simulink model "slip_model_Student"  (Simulink 8.7)
settings: Solver=ode45  StartTime=0.0  StopTime=20  RelTol=1e-3
values from neighbouring files (symbols this model uses):
  AA = [0 1 0 0 0 0; -Veh.kc/Veh.mc -Veh.cc/Veh.mc Veh.kc/Veh.mc Veh.cc/Veh.mc 0 0; 0 0 0 1 0 0; Veh.kc/Veh.mb Veh.cc/Veh.mb -(Veh.kc+Veh.kb)/Veh.mb -(Veh.cc+Veh.cb)/Veh.mb Veh.kb/Veh.mb Veh.cb/Veh.mb; 0 0 0 0 1 0; 0 0 Veh.kb/Veh.mw Veh.cb/Veh.mw -(Veh.kb+Veh.kw)/Veh.mw -(Veh.cb+Veh.cw)/Veh.mw]    [initial.m]
  BB = [0 0; 0 0; 0 0; 0 0; 0 0; Veh.kw/Veh.mw Veh.cw/Veh.mw]    [initial.m]
  CC = [0 0 0 0 -Veh.kw -Veh.cw]    [initial.m]
  DD = [Veh.kw Veh.cw]    [initial.m]
  k_b = 0.6    [Task2b.m]    (also in Task2bLooping.m; Task2c.m = 1; initial.m = 0.2)
  k_t = 0    [Task2b.m]    (also in Task2bLooping.m; Task2c.m = 0.7356; initial.m = 0.23)
  T_max = (Veh.mc+Veh.mb+Veh.mw)*9.81*Veh.r    [initial.m]
undefined symbols (not defined in the file or in its folder): Dri, Veh
libraries: driveline x8, simulink x2
settings Model: Creator=Johannes  LastModifiedBy=Dell
settings DataIOCC: LimitDataPoints=off
settings OptimizationCC: ExpressionDepthLimit=2147483647
settings DebuggingCC: SolverPrmCheckMsg=warning  FcnCallInpInsideContextMsg=UseLocalSettings  StateNameClashWarn=warning
settings GRTTargetCC: CombineOutputUpdateFcns=off  GRTInterface=on

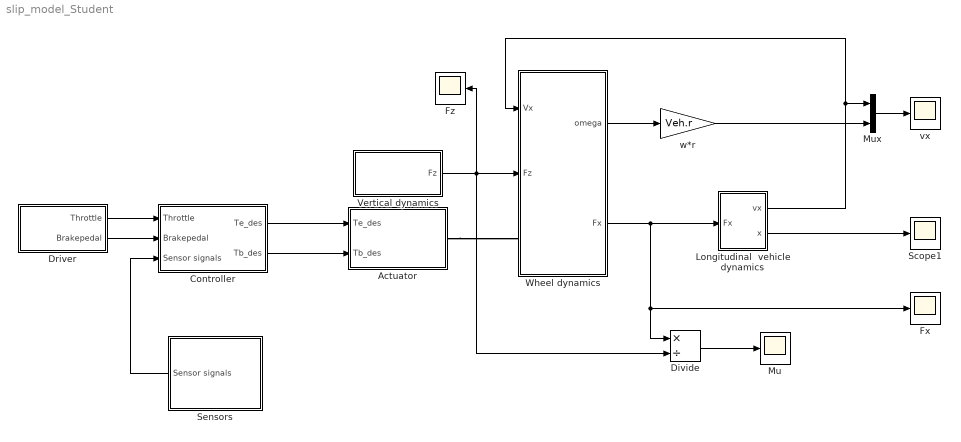
== system slip_model_Student ==
  Actuator : Subsystem
  Controller : Subsystem
  Divide : Product  Inputs=*/
  Driver : Subsystem
  Fx : Scope
  Fz : Scope
  Longitudinal  vehicle dynamics : Subsystem
  "Mu " : Scope
  Mux : Mux  Inputs=2
  Scope1 : Scope
  Sensors : Subsystem
  Vertical dynamics : Subsystem
  Wheel dynamics : Subsystem
  vx : Scope
  w*r : Gain  Gain=Veh.r
  wires:
  Longitudinal  vehicle dynamics/2(x) -> Scope1/1
  Mux/1 -> vx/1
  w*r/1 -> Mux/2
  Wheel dynamics/1(omega) -> w*r/1
  Wheel dynamics/2(Fx) -> Longitudinal  vehicle dynamics/1(Fx), Divide/1, Fx/1
  Vertical dynamics/1(Fz) -> Fz/1, Divide/2, Wheel dynamics/2(Fz)
  Driver/2(Brakepedal) -> Controller/2(Brakepedal)
  Driver/1(Throttle) -> Controller/1(Throttle)
  Controller/1(Te_des) -> Actuator/1(Te_des)
  Controller/2(Tb_des) -> Actuator/2(Tb_des)
  Sensors/1(Sensor signals) -> Controller/3(Sensor signals)
  Longitudinal  vehicle dynamics/1(vx) -> Mux/1, Wheel dynamics/1(Vx)
  Divide/1 -> "Mu "/1
  connections:
  Actuator/RConn1 -- Wheel dynamics/LConn1

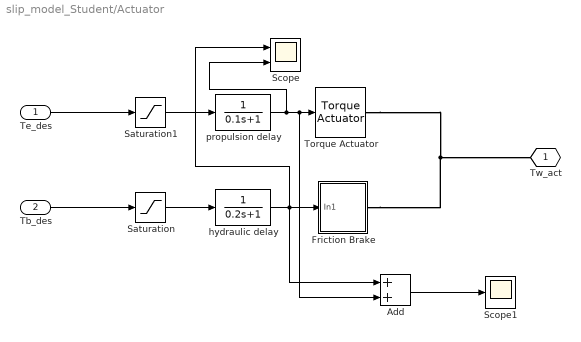
== system slip_model_Student/Actuator ==
  Te_des : Inport
  Tb_des : Inport  Port=2
  Add : Sum
  Friction Brake : Subsystem
  Saturation : Saturate  UpperLimit=0  LowerLimit=-inf
  Saturation1 : Saturate  UpperLimit=inf  LowerLimit=0
  Scope : Scope  NumInputPorts=2
  Scope1 : Scope
  Torque Actuator : driveline/Sensors & Actuators/Torque Actuator
  hydraulic delay : TransferFcn  Denominator=[0.2 1]
  propulsion delay : TransferFcn  Denominator=[0.1 1]
  Tw_act : PMIOPort  Tag=PMCPort  Port=1  Side=Right
  wires:
  Te_des/1 -> Saturation1/1
  Tb_des/1 -> Saturation/1
  propulsion delay/1 -> Add/2, Torque Actuator/1, Scope/2
  Saturation1/1 -> propulsion delay/1
  Saturation/1 -> hydraulic delay/1
  hydraulic delay/1 -> Add/1, Scope/1, Friction Brake/1(In1)
  Add/1 -> Scope1/1
  connections:
  Friction Brake/RConn1 -- Torque Actuator/RConn1 -- Tw_act/RConn1

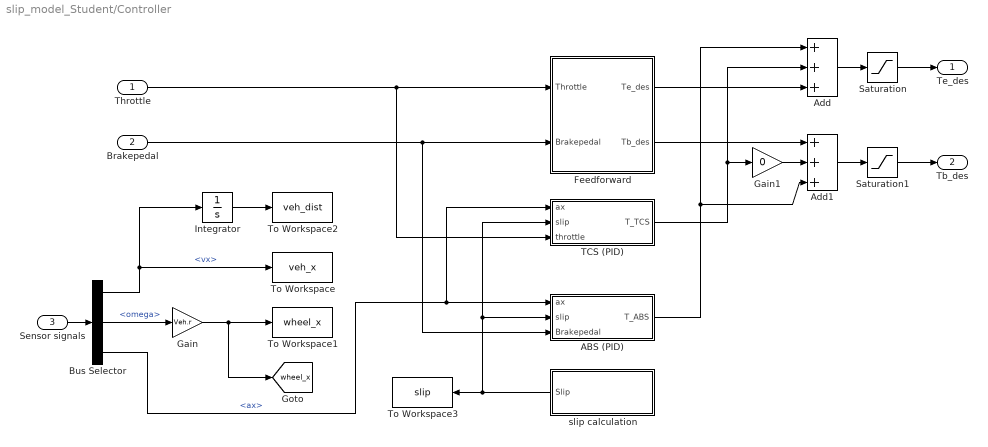
== system slip_model_Student/Controller ==
  Throttle : Inport
  Brakepedal : Inport  Port=2
  Sensor signals : Inport  Port=3
  ABS (PID) : Subsystem
  Add : Sum  Inputs=+++
  Add1 : Sum  Inputs=+++
  Bus Selector : BusSelector  OutputSignals=vx,omega,ax
  Feedforward : Subsystem
  Gain : Gain  Gain=Veh.r
  Gain1 : Gain  Gain=0
  Integrator : Integrator
  Saturation : Saturate  UpperLimit=T_max  LowerLimit=0
  Saturation1 : Saturate  UpperLimit=0  LowerLimit=-T_max
  TCS (PID) : Subsystem
  To Workspace : ToWorkspace  VariableName=veh_x  SaveFormat=Timeseries  SampleTime=-1
  To Workspace1 : ToWorkspace  VariableName=wheel_x  SaveFormat=Timeseries  SampleTime=-1
  To Workspace2 : ToWorkspace  VariableName=veh_dist  SaveFormat=Timeseries  SampleTime=-1
  To Workspace3 : ToWorkspace  VariableName=slip  SaveFormat=Timeseries  SampleTime=-1
  slip calculation : Subsystem
  Te_des : Outport
  Tb_des : Outport  Port=2
  tag scope: wheel_x=global
  wires:
  Throttle/1 -> TCS (PID)/3(throttle), Feedforward/1(Throttle)
  Brakepedal/1 -> ABS (PID)/3("Brakepedal "), Feedforward/2(Brakepedal)
  Sensor signals/1 -> Bus Selector/1
  Bus Selector/2 -> Gain/1  "<omega>"
  Bus Selector/1 -> To Workspace/1, Integrator/1  "<vx>"
  Gain/1 -> [wheel_x], To Workspace1/1
  Integrator/1 -> To Workspace2/1
  slip calculation/1(Slip) -> TCS (PID)/2(slip), ABS (PID)/2(slip), To Workspace3/1
  Bus Selector/3 -> TCS (PID)/1(ax), ABS (PID)/1(ax)  "<ax>"
  Add1/1 -> Saturation1/1
  Feedforward/2(Tb_des) -> Add1/1
  TCS (PID)/1(T_TCS) -> Gain1/1, Add/2
  ABS (PID)/1(T_ABS) -> Add1/3, Add/1
  Add/1 -> Saturation/1
  Saturation/1 -> Te_des/1
  Saturation1/1 -> Tb_des/1
  Gain1/1 -> Add1/2
  Feedforward/1(Te_des) -> Add/3

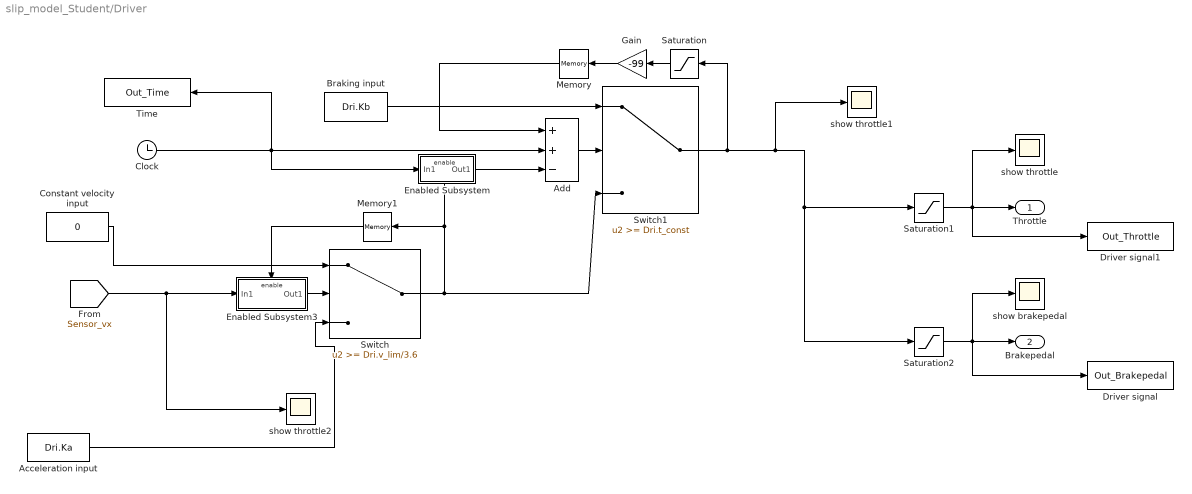
== system slip_model_Student/Driver ==
  Acceleration input : Constant  Value=Dri.Ka
  Add : Sum  Inputs=++-
  Braking input : Constant  Value=Dri.Kb
  Clock : Clock
  Constant velocity input : Constant  Value=0
  Driver signal : ToWorkspace  VariableName=Out_Brakepedal  SampleTime=-1
  Driver signal1 : ToWorkspace  VariableName=Out_Throttle  SampleTime=-1
  Enabled Subsystem : Subsystem  TreatAsAtomicUnit=on
  Enabled Subsystem3 : Subsystem  TreatAsAtomicUnit=on
  Gain : Gain  Gain=-99
  Memory : Memory
  Memory1 : Memory
  Saturation : Saturate  UpperLimit=0  LowerLimit=-1
  Saturation1 : Saturate  UpperLimit=1  LowerLimit=0
  Saturation2 : Saturate  UpperLimit=0  LowerLimit=-1
  Switch : Switch  Threshold=Dri.v_lim/3.6
  Switch1 : Switch  Threshold=Dri.t_const
  Time : ToWorkspace  VariableName=Out_Time  SampleTime=-1
  show brakepedal : Scope
  show throttle : Scope
  show throttle1 : Scope
  show throttle2 : Scope
  Throttle : Outport
  Brakepedal : Outport  Port=2
  wires:
  Constant velocity input/1 -> Switch/1
  Braking input/1 -> Switch1/1
  Clock/1 -> Add/2, Time/1, Enabled Subsystem/1(In1)
  Add/1 -> Switch1/2
  Switch/1 -> Switch1/3, Enabled Subsystem/Enable, Memory1/1
  Switch1/1 -> Saturation/1, Saturation1/1, Saturation2/1, show throttle1/1
  Enabled Subsystem/1(Out1) -> Add/3
  Saturation/1 -> Gain/1
  Gain/1 -> Memory/1
  Memory/1 -> Add/1
  [Sensor_vx] -> Enabled Subsystem3/1(In1), show throttle2/1
  Enabled Subsystem3/1(Out1) -> Switch/2
  Memory1/1 -> Enabled Subsystem3/Enable
  Saturation1/1 -> Throttle/1, Driver signal1/1, show throttle/1
  Saturation2/1 -> Brakepedal/1, Driver signal/1, show brakepedal/1
  Acceleration input/1 -> Switch/3

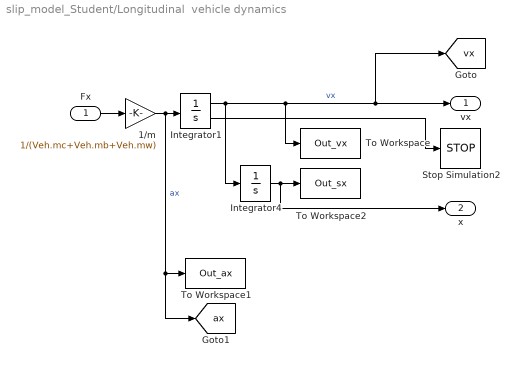
== system slip_model_Student/Longitudinal  vehicle dynamics ==
  Fx : Inport
  1/m : Gain  Gain=1/(Veh.mc+Veh.mb+Veh.mw)
  Integrator1 : Integrator  LowerSaturationLimit=0.0  ShowSaturationPort=on
  Integrator4 : Integrator  InitialCondition=0.01  LimitOutput=on  LowerSaturationLimit=0.0
  Stop Simulation2 : Stop
  To Workspace : ToWorkspace  VariableName=Out_vx  SampleTime=-1
  To Workspace1 : ToWorkspace  VariableName=Out_ax  SampleTime=-1
  To Workspace2 : ToWorkspace  VariableName=Out_sx  SampleTime=-1
  vx : Outport
  x : Outport  Port=2
  tag scope: ax=global, vx=global
  wires:
  1/m/1 -> Integrator1/1, [ax], To Workspace1/1  "ax"
  Integrator1/1 -> To Workspace/1, vx/1, [vx], Integrator4/1  "vx"
  Integrator4/1 -> To Workspace2/1, x/1
  Fx/1 -> 1/m/1
  Integrator1/2 -> Stop Simulation2/1

== system slip_model_Student/Sensors ==
  Bus Creator : BusCreator  Inputs=3
  Sensor signals : Outport
  tag scope: Sensor_vx=global
  wires:
  [vx] -> Bus Creator/1, [Sensor_vx]
  [omega] -> Bus Creator/2
  Bus Creator/1 -> Sensor signals/1
  [ax] -> Bus Creator/3

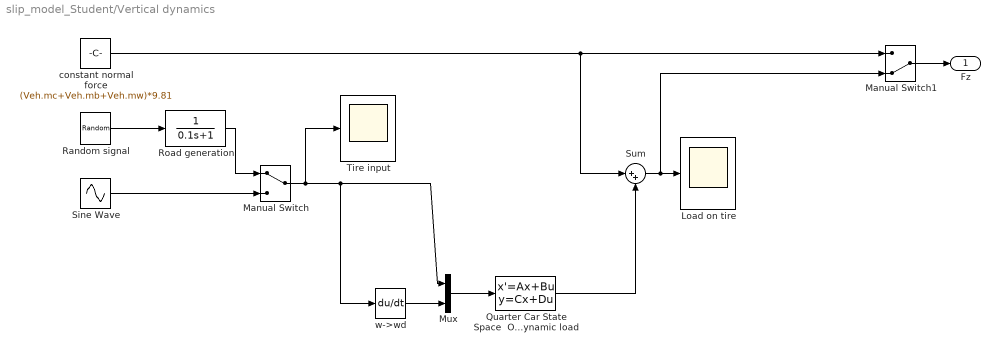
== system slip_model_Student/Vertical dynamics ==
  Load on tire : Scope
  Manual Switch : ManualSwitch
  Manual Switch1 : ManualSwitch  CurrentSetting=0
  Mux : Mux  Inputs=2
  Quarter Car State Space  Output: dynamic load : StateSpace  A=AA  B=BB  C=CC  D=DD  X0=[0 0 0 0 0 0]
  Random signal : UniformRandomNumber  Minimum=-0.01  Maximum=0.01  SampleTime=0.001
  Road generation : TransferFcn  Denominator=[0.1 1]
  Sine Wave : Sin  Amplitude=0.01  Frequency=12*2*pi  SampleTime=0
  Sum : Sum  Inputs=|++
  Tire input : Scope
  constant normal force : Constant  Value=(Veh.mc+Veh.mb+Veh.mw)*9.81
  w->wd : Derivative
  Fz : Outport
  wires:
  Random signal/1 -> Road generation/1
  w->wd/1 -> Mux/2
  Quarter Car State Space  Output: dynamic load/1 -> Sum/2
  Mux/1 -> Quarter Car State Space  Output: dynamic load/1
  Sine Wave/1 -> Manual Switch/2
  Manual Switch/1 -> w->wd/1, Mux/1, Tire input/1
  constant normal force/1 -> Manual Switch1/1, Sum/1
  Manual Switch1/1 -> Fz/1
  Sum/1 -> Load on tire/1, Manual Switch1/2
  Road generation/1 -> Manual Switch/1

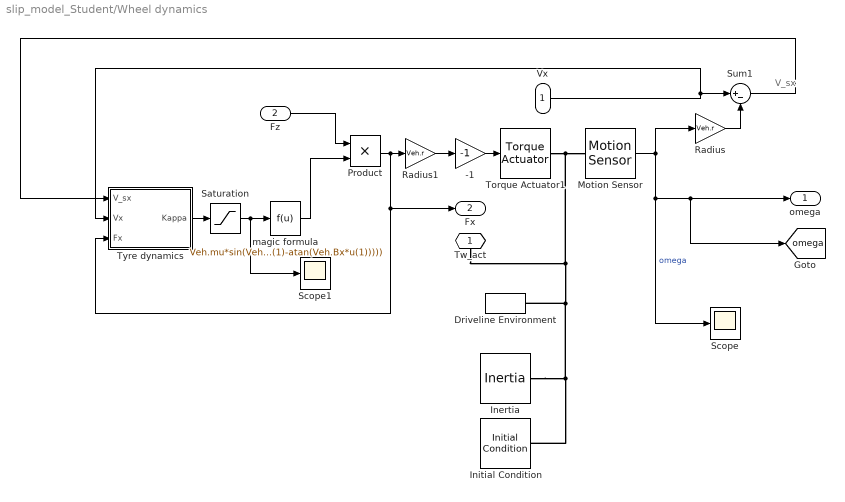
== system slip_model_Student/Wheel dynamics ==
  note: V_sx
  Vx : Inport
  Fz : Inport  Port=2
  -1 : Gain  Gain=-1
  Driveline Environment : driveline/Solver & Inertias/Driveline Environment  PortType=p1  BlockClass=Solver  PhysicalDomain=driveline_domain  SimulationMode=Dynamics  ModeIteration=off  DefaultClutchVelocityTolerance=1e-3  DefaultUseAutoClutchVelocityTolerance=on
  Inertia : driveline/Solver & Inertias/Inertia  PortType=p1  BlockClass=Inertia  PhysicalDomain=driveline_domain  I=Veh.Jw  Ip=[]  Iv=[]  ShowLeft=off  ShowRight=on
  Initial Condition : driveline/Sensors & Actuators/Initial Condition  PortType=p1  BlockClass=Inertia  PhysicalDomain=driveline_domain  I=0  Ip=[]  Iv=0  ShowLeft=off  ShowRight=on
  Motion Sensor : driveline/Sensors & Actuators/Motion Sensor  Angle=off  x0=0  Velocity=on  Acceleration=off
  Product : Product  RndMeth=Zero
  Radius : Gain  Gain=Veh.r
  Radius1 : Gain  Gain=Veh.r
  Saturation : Saturate  UpperLimit=1  LowerLimit=-1
  Scope : Scope
  Scope1 : Scope
  Sum1 : Sum  Inputs=|+-
  Torque Actuator1 : driveline/Sensors & Actuators/Torque Actuator
  Tyre dynamics : Subsystem
  magic formula : Fcn  Expr=Veh.mu*sin(Veh.Cx*atan(Veh.Bx*u(1)-Veh.Ex*(Veh.Bx*u(1)-atan(Veh.Bx*u(1)))))
  Tw_act : PMIOPort  Port=1  Side=Left
  omega : Outport
  Fx : Outport  Port=2
  tag scope: omega=global
  wires:
  Radius/1 -> Sum1/2
  Vx/1 -> Tyre dynamics/2(Vx), Sum1/1
  Motion Sensor/1 -> Radius/1, Scope/1, omega/1, [omega]  "omega"
  -1/1 -> Torque Actuator1/1
  Radius1/1 -> -1/1
  magic formula/1 -> Product/2
  Product/1 -> Radius1/1, Tyre dynamics/3(Fx), Fx/1
  Sum1/1 -> Tyre dynamics/1(V_sx)
  Fz/1 -> Product/1
  Tyre dynamics/1(Kappa) -> Saturation/1
  Saturation/1 -> magic formula/1, Scope1/1
  connections:
  Initial Condition/RConn1 -- Torque Actuator1/RConn1 -- Motion Sensor/LConn1 -- Tw_act/RConn1 -- Driveline Environment/LConn1 -- Inertia/RConn1

== system slip_model_Student/Actuator/Friction Brake ==
  In1 : Inport
  Controllable Friction Clutch : driveline/Dynamic Elements/Controllable Friction Clutch  Sign=Unidirectional  Nf=1  EffectiveRadius=0.1  PeakForce=1000  MuTable=[0 1; 1e8 1]  PeakFactor=1.1  PressureEngagementThreshold=0  UseDefaultVelocityTolerance=on  VelocityTolerance=1e-3  UseAutomaticVelocityTolerance=on  Lock=off  Slip=off  EnergyLoss=off  Mode=off  SimDrivelineLibraryVersion=1.1  BlockClass=Clutch
  Housing : driveline/Solver & Inertias/Housing
  Rate Limiter : RateLimiter  RisingSlewLimit=25000*Veh.r  FallingSlewLimit=-83000*Veh.r  SampleTimeMode=inherited
  w*r : Gain  Gain=0.01
  w*r1 : Gain  Gain=-1
  shaft : PMIOPort  Port=1  Side=Right
  wires:
  In1/1 -> w*r1/1
  Rate Limiter/1 -> Controllable Friction Clutch/1
  w*r/1 -> Rate Limiter/1
  w*r1/1 -> w*r/1
  connections:
  Housing/RConn1 -- Controllable Friction Clutch/LConn1
  shaft/RConn1 -- Controllable Friction Clutch/RConn1

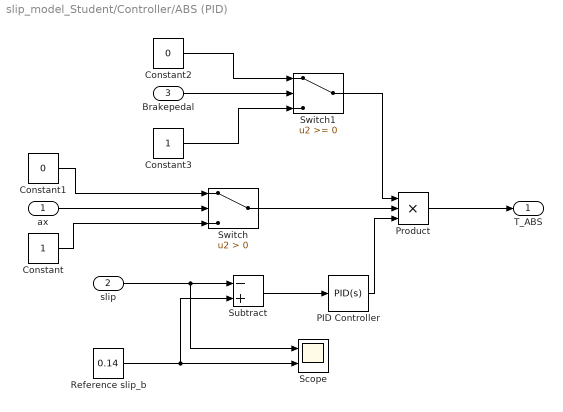
== system slip_model_Student/Controller/ABS (PID) ==
  ax : Inport
  slip : Inport  Port=2
  "Brakepedal " : Inport  Port=3
  Constant : Constant
  Constant1 : Constant  Value=0
  Constant2 : Constant  Value=0
  Constant3 : Constant
  PID Controller : simulink/Continuous/PID Controller  Controller=PID  TimeDomain=Continuous-time  SampleTime=-1  IntegratorMethod=Forward Euler  FilterMethod=Forward Euler  Form=Parallel  UseFilter=on  ControllerParametersSource=internal  P=-18000  I=-1  D=-350  N=100  InitialConditionSource=internal  InitialConditionForIntegrator=0  InitialConditionForFilter=0  ExternalReset=none  LimitOutput=off  UpperSaturationLimit=inf  LowerSaturationLimit=-inf  LinearizeAsGain=on  AntiWindupMode=none  Kb=1  TrackingMode=off  Kt=1  PParamMin=[]  PParamMax=[]  IParamMin=[]  IParamMax=[]  DParamMin=[]  DParamMax=[]  NParamMin=[]  NParamMax=[]  KbParamMin=[]  KbParamMax=[]  KtParamMin=[]  KtParamMax=[]  POutMin=[]  POutMax=[]  IOutMin=[]  IOutMax=[]  DOutMin=[]  DOutMax=[]  NOutMin=[]  NOutMax=[]  KbOutMin=[]  KbOutMax=[]  KtOutMin=[]  KtOutMax=[]  IntegratorOutMin=[]  IntegratorOutMax=[]  FilterOutMin=[]  FilterOutMax=[]  SumOutMin=[]  SumOutMax=[]  SumI1OutMin=[]  SumI1OutMax=[]  SumI2OutMin=[]  SumI2OutMax=[]  SumI3OutMin=[]  SumI3OutMax=[]  SumDOutMin=[]  SumDOutMax=[]  SaturationOutMin=[]  SaturationOutMax=[]  IntegratorContinuousStateAttributes=''  IntegratorStateMustResolveToSignalObject=off  IntegratorRTWStateStorageClass=Auto  FilterContinuousStateAttributes=''  FilterStateMustResolveToSignalObject=off  FilterRTWStateStorageClass=Auto  DifferentiatorICPrevScaledInput=0  DifferentiatorOutMin=[]  DifferentiatorOutMax=[]
  Product : Product  Inputs=3
  Reference slip_b : Constant  Value=0.14
  Scope : Scope  NumInputPorts=2
  Subtract : Sum  Inputs=-+
  Switch : Switch  Criteria=u2 > Threshold
  Switch1 : Switch
  T_ABS : Outport
  wires:
  slip/1 -> Scope/1, Subtract/1
  Reference slip_b/1 -> Scope/2, Subtract/2
  Subtract/1 -> PID Controller/1
  ax/1 -> Switch/2
  Switch/1 -> Product/2
  PID Controller/1 -> Product/3
  Product/1 -> T_ABS/1
  Constant1/1 -> Switch/1
  Constant/1 -> Switch/3
  "Brakepedal "/1 -> Switch1/2
  Constant2/1 -> Switch1/1
  Constant3/1 -> Switch1/3
  Switch1/1 -> Product/1

== system slip_model_Student/Controller/Feedforward ==
  Throttle : Inport
  Brakepedal : Inport  Port=2
  Gain : Gain  Gain=k_t*T_max
  Gain1 : Gain  Gain=k_b*T_max
  Scope : Scope
  Te_des : Outport
  Tb_des : Outport  Port=2
  wires:
  Throttle/1 -> Scope/1, Gain/1
  Brakepedal/1 -> Gain1/1
  Gain/1 -> Te_des/1
  Gain1/1 -> Tb_des/1

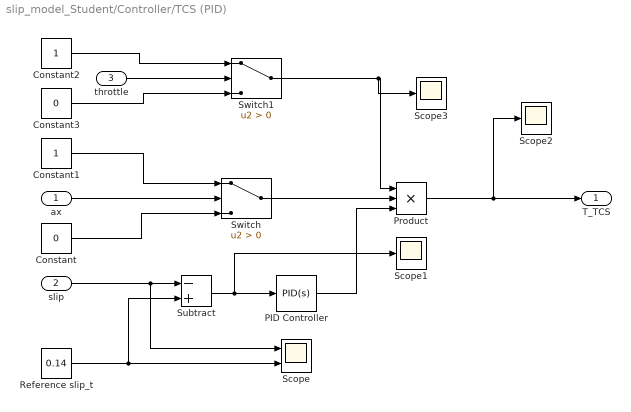
== system slip_model_Student/Controller/TCS (PID) ==
  ax : Inport
  slip : Inport  Port=2
  throttle : Inport  Port=3
  Constant : Constant  Value=0
  Constant1 : Constant
  Constant2 : Constant
  Constant3 : Constant  Value=0
  PID Controller : simulink/Continuous/PID Controller  Controller=PID  TimeDomain=Continuous-time  SampleTime=-1  IntegratorMethod=Forward Euler  FilterMethod=Forward Euler  Form=Parallel  UseFilter=on  ControllerParametersSource=internal  P=20000  I=200  D=1500  N=1000  InitialConditionSource=internal  InitialConditionForIntegrator=0  InitialConditionForFilter=0  ExternalReset=none  LimitOutput=off  UpperSaturationLimit=inf  LowerSaturationLimit=-inf  LinearizeAsGain=on  AntiWindupMode=none  Kb=1  TrackingMode=off  Kt=1  PParamMin=[]  PParamMax=[]  IParamMin=[]  IParamMax=[]  DParamMin=[]  DParamMax=[]  NParamMin=[]  NParamMax=[]  KbParamMin=[]  KbParamMax=[]  KtParamMin=[]  KtParamMax=[]  POutMin=[]  POutMax=[]  IOutMin=[]  IOutMax=[]  DOutMin=[]  DOutMax=[]  NOutMin=[]  NOutMax=[]  KbOutMin=[]  KbOutMax=[]  KtOutMin=[]  KtOutMax=[]  IntegratorOutMin=[]  IntegratorOutMax=[]  FilterOutMin=[]  FilterOutMax=[]  SumOutMin=[]  SumOutMax=[]  SumI1OutMin=[]  SumI1OutMax=[]  SumI2OutMin=[]  SumI2OutMax=[]  SumI3OutMin=[]  SumI3OutMax=[]  SumDOutMin=[]  SumDOutMax=[]  SaturationOutMin=[]  SaturationOutMax=[]  IntegratorContinuousStateAttributes=''  IntegratorStateMustResolveToSignalObject=off  IntegratorRTWStateStorageClass=Auto  FilterContinuousStateAttributes=''  FilterStateMustResolveToSignalObject=off  FilterRTWStateStorageClass=Auto  DifferentiatorICPrevScaledInput=0  DifferentiatorOutMin=[]  DifferentiatorOutMax=[]
  Product : Product  Inputs=3
  Reference slip_t : Constant  Value=0.14
  Scope : Scope  NumInputPorts=2
  Scope1 : Scope
  Scope2 : Scope
  Scope3 : Scope
  Subtract : Sum  Inputs=-+
  Switch : Switch  Criteria=u2 > Threshold
  Switch1 : Switch  Criteria=u2 > Threshold
  T_TCS : Outport
  wires:
  Reference slip_t/1 -> Scope/2, Subtract/2
  Subtract/1 -> Scope1/1, PID Controller/1
  ax/1 -> Switch/2
  Switch/1 -> Product/2
  PID Controller/1 -> Product/3
  Product/1 -> Scope2/1, T_TCS/1
  Constant1/1 -> Switch/1
  Constant/1 -> Switch/3
  Constant2/1 -> Switch1/1
  Constant3/1 -> Switch1/3
  slip/1 -> Scope/1, Subtract/1
  Switch1/1 -> Scope3/1, Product/1
  throttle/1 -> Switch1/2

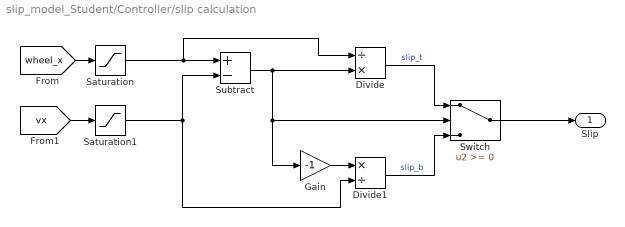
== system slip_model_Student/Controller/slip calculation ==
  Divide : Product  Inputs=/*
  Divide1 : Product  Inputs=*/
  Gain : Gain  Gain=-1
  Saturation : Saturate  UpperLimit=inf  LowerLimit=0.001
  Saturation1 : Saturate  UpperLimit=inf  LowerLimit=0.001
  Subtract : Sum  Inputs=+-
  Switch : Switch
  Slip : Outport
  wires:
  [wheel_x] -> Saturation/1
  Subtract/1 -> Divide/2, Switch/2, Gain/1
  Gain/1 -> Divide1/1
  Divide/1 -> Switch/1  "slip_t"
  Divide1/1 -> Switch/3  "slip_b"
  [vx] -> Saturation1/1
  Switch/1 -> Slip/1
  Saturation/1 -> Divide/1, Subtract/1
  Saturation1/1 -> Subtract/2, Divide1/2

== system slip_model_Student/Driver/Enabled Subsystem ==
  In1 : Inport
  Enable : EnablePort
  Out1 : Outport
  wires:
  In1/1 -> Out1/1

== system slip_model_Student/Driver/Enabled Subsystem3 ==
  In1 : Inport
  Enable : EnablePort  StatesWhenEnabling=reset  PropagateVarSize=During execution
  Out1 : Outport
  wires:
  In1/1 -> Out1/1

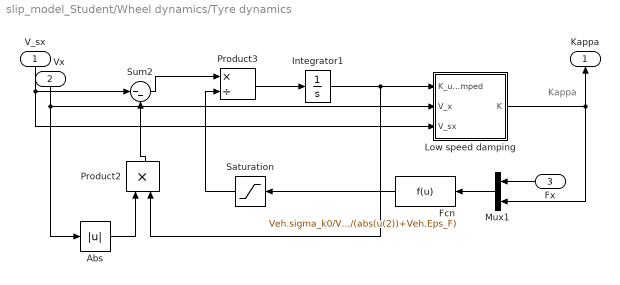
== system slip_model_Student/Wheel dynamics/Tyre dynamics ==
  note: Kappa
  V_sx : Inport
  Vx : Inport  Port=2
  Fx : Inport  Port=3
  Abs : Abs
  Fcn : Fcn  Expr=Veh.sigma_k0/Veh.C_fk*(abs(u(1))+Veh.C_fk*Veh.Eps_F)/(abs(u(2))+Veh.Eps_F)
  Integrator1 : Integrator
  Low speed damping : Subsystem
  Mux1 : Mux  Inputs=2
  Product2 : Product  RndMeth=Zero
  Product3 : Product  Inputs=*/  RndMeth=Zero
  Saturation : Saturate  UpperLimit=Inf  LowerLimit=Veh.sigma_min
  Sum2 : Sum  Inputs=|--
  Kappa : Outport
  wires:
  Sum2/1 -> Product3/1
  Low speed damping/1(K) -> Mux1/2, Kappa/1
  Abs/1 -> Product2/1
  Product2/1 -> Sum2/2
  Saturation/1 -> Product3/2
  Mux1/1 -> Fcn/1
  Product3/1 -> Integrator1/1
  Integrator1/1 -> Low speed damping/1(K_undamped), Product2/2
  Fcn/1 -> Saturation/1
  V_sx/1 -> Sum2/1, Low speed damping/3(V_sx)
  Vx/1 -> Low speed damping/2(V_x), Abs/1
  Fx/1 -> Mux1/1

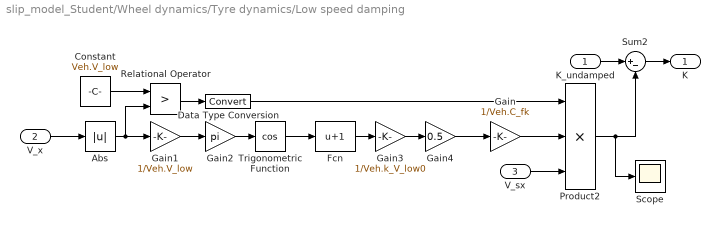
== system slip_model_Student/Wheel dynamics/Tyre dynamics/Low speed damping ==
  K_undamped : Inport
  V_x : Inport  Port=2
  V_sx : Inport  Port=3
  Abs : Abs
  Constant : Constant  Value=Veh.V_low
  Data Type Conversion : DataTypeConversion  RndMeth=Zero
  Fcn : Fcn  Expr=u+1
  Gain : Gain  Gain=1/Veh.C_fk
  Gain1 : Gain  Gain=1/Veh.V_low
  Gain2 : Gain  Gain=pi
  Gain3 : Gain  Gain=1/Veh.k_V_low0
  Gain4 : Gain  Gain=0.5
  Product2 : Product  Inputs=3  RndMeth=Zero
  Relational Operator : RelationalOperator  Operator=>  OutDataTypeStr=boolean
  Scope : Scope
  Sum2 : Sum  Inputs=|+-
  Trigonometric Function : Trigonometry  Operator=cos
  K : Outport
  wires:
  Product2/1 -> Sum2/2, Scope/1
  Constant/1 -> Relational Operator/1
  Abs/1 -> Relational Operator/2, Gain1/1
  Relational Operator/1 -> Data Type Conversion/1
  Data Type Conversion/1 -> Product2/1
  Gain1/1 -> Gain2/1
  Gain2/1 -> Trigonometric Function/1
  Trigonometric Function/1 -> Fcn/1
  Fcn/1 -> Gain3/1
  Gain3/1 -> Gain4/1
  Gain4/1 -> Gain/1
  Gain/1 -> Product2/2
  V_x/1 -> Abs/1
  V_sx/1 -> Product2/3
  K_undamped/1 -> Sum2/1
  Sum2/1 -> K/1
